simulink model "generate_joint_velocity_motion"  (R2019a)
settings: Solver=FixedStepDiscrete  StartTime=0.0  StopTime=inf  FixedStep=0.001  RelTol=1e-3  EnableMultiTasking=on
PreLoadFcn:
  | demos_common_configs();
undefined symbols (not defined in the file): DiscIntNeverNeededParam
libraries: franka_simulink_library_misc x5, franka_simulink_library x3
settings Model: SimulationMode=external  ExtModeTrigDuration=10000  Creator=vasi_ko  LastModifiedBy=kvasios
settings DataIOCC: LimitDataPoints=on  SaveFormat=Array  ReturnWorkspaceOutputs=off
settings OptimizationCC: DefaultParameterBehavior=Inlined  EnhancedBackFolding=on  PassReuseOutputArgsAs=Individual arguments  ZeroExternalMemoryAtStartup=off  ZeroInternalMemoryAtStartup=off  OptimizeBlockOrder=speed  DifferentSizesBufferReuse=on  OptimizationCustomize=off
settings DebuggingCC: SolverPrmCheckMsg=warning  ParameterTunabilityLossMsg=error  SFUnexpectedBacktrackingDiag=warning  SFNoUnconditionalDefaultTransitionDiag=warning  SFExecutionAtInitializationDiag=none  ArithmeticOperatorsInVariantConditions=warning
settings HardwareCC: ProdBitPerLong=64  ProdHWDeviceType=Intel->x86-64 (Linux 64)
settings ModelReferenceCC: PropagateSignalLabelsOutOfModel=off
settings SFSimCC: SimUseLocalCustomCode=off  MATLABDynamicMemAlloc=off
settings RTWCC: SystemTargetFile=franka_emika_panda.tlc  GenCodeOnly=on  TemplateMakefile=ert_default_tmf  RTWVerbose=off  RTWUseLocalCustomCode=off  Toolchain=Franka Simulink | gmake (64-bit linux)  BuildConfiguration=Faster Runs  IncludeHyperlinkInReport=on  TargetLang=C++
settings CodeAppCC: ForceParamTrailComments=on  IgnoreCustomStorageClasses=off  OperatorAnnotations=on  SimulinkDataObjDesc=on  SFDataObjDesc=on  InsertBlockDesc=on
settings STFCustomTargetCC: TargetLangStandard=C99 (ISO)  MultiwordLength=256  GenerateSampleERTMain=on  ModelReferenceCompliant=off  CombineOutputUpdateFcns=on  ERTCustomFileBanners=on  SupportNonInlinedSFcns=off  RemoveResetFunc=on  MATLABClassNameForMDSCustomization=Simulink.SoftwareTarget.ERTCustomization  CPPClassGenCompliant=on  GRTInterface=off  UseToolchainInfoCompliant=on  SystemTargetFile=franka_emika_panda.tlc
settings ERTTargetCC: TargetLangStandard=C99 (ISO)  GenerateSampleERTMain=on  ModelReferenceCompliant=off  ParMdlRefBuildCompliant=off  CompOptLevelCompliant=off  ConcurrentExecutionCompliant=off  SupportContinuousTime=on  ModelStepFunctionPrototypeControlCompliant=off  InlinedParameterPlacement=NonHierarchical  ERTCustomFileTemplate=franka_emika_panda_file_process.tlc
settings ConfigComp: CovMetricSettings=dw  CovSaveCumulativeToWorkspaceVar=on  CovSaveSingleToWorkspaceVar=on  CovExternalEMLEnable=off  CovSFcnEnable=off

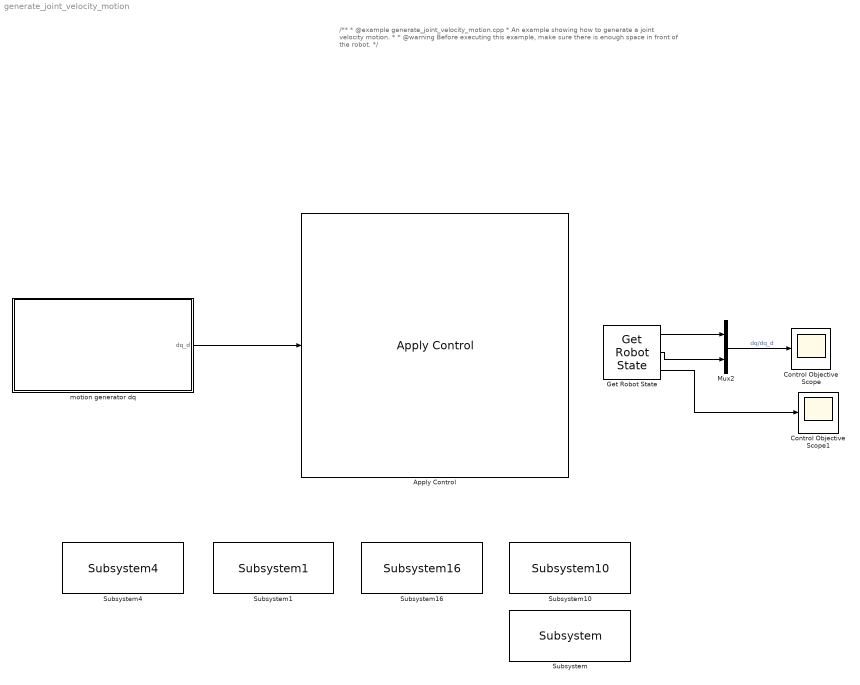
== system generate_joint_velocity_motion ==
  note: /**
      |  * @example generate_joint_velocity_motion.cpp
      |  * An example showing how to generate a joint velocity motion.
      |  *
      |  * @warning Before executing this example, make sure there is enough space in front of the robot.
      |  */
  Apply Control : franka_simulink_library/Apply Control  robot_ip=robot_ip  gripper_attached=off  control_mode=Joint Velocities - Internal Controller Mode  controller_choice=Joint Impedance Controller  elbow_control=on  collision_thresholds=collision_behavior  joint_impedance=joint_impedance  cartesian_impedance=cartesian_impedance  load_inertia=load_inertia  EE_T_K=EE_T_K  init_joint_configuration_req=on  init_joint_configuration=[0, -pi/4, 0, -3 * pi/4, 0, pi/2, pi/4]
      settings: SourceProductName=Franka Emika
  Control Objective Scope : Scope
  Control Objective Scope1 : Scope
  Get Robot State : franka_simulink_library/Get Robot State  robot_ip=robot_ip  signals_requested='dq dq_d control_command_success_rate'
      settings: SourceProductName=Franka Emika
  Mux2 : Mux  Inputs=2
  Subsystem : franka_simulink_library_misc/Subsystem  SystemSampleTime=-1  Latency=0  AutoFrameSizeCalculation=off
  Subsystem1 : franka_simulink_library_misc/Subsystem1  SystemSampleTime=-1  Latency=0  AutoFrameSizeCalculation=off
  Subsystem10 : franka_simulink_library_misc/Subsystem10  SystemSampleTime=-1  Latency=0  AutoFrameSizeCalculation=off
  Subsystem16 : franka_simulink_library_misc/Subsystem16  SystemSampleTime=-1  Latency=0  AutoFrameSizeCalculation=off
  Subsystem4 : franka_simulink_library_misc/Subsystem4  SystemSampleTime=-1  Latency=0  AutoFrameSizeCalculation=off
  motion generator dq : Subsystem
      mask Display:
      | pos = get_param(gcb, 'Position');
      | width = pos(3) - pos(1);
      | x = [0:width];
      | y = sin(x/180*pi);
      | % Parameters 'm' and 'b' must be defined in 'Parameters & Dialog' pane.
      | plot(x,y );
      | 
      | port_label('output',1,'dq_d');
  wires:
  Get Robot State/1 -> Mux2/1
  Get Robot State/2 -> Mux2/2
  Mux2/1 -> Control Objective Scope/1  "dq/dq_d"
  motion generator dq/1(dq_d) -> Apply Control/1
  Get Robot State/3 -> Control Objective Scope1/1

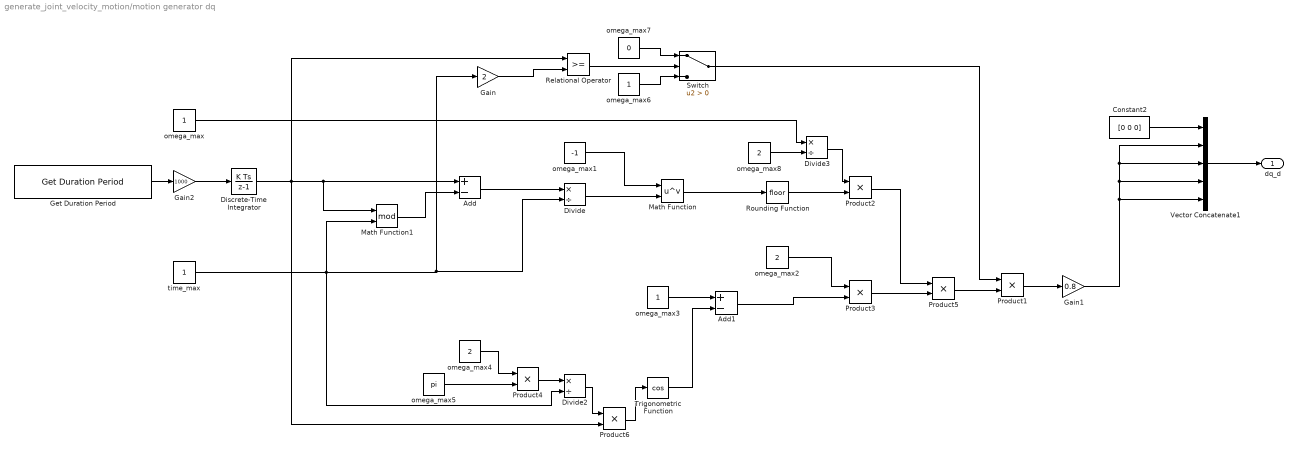
== system generate_joint_velocity_motion/motion generator dq ==
  Add : Sum  Inputs=+-
  Add1 : Sum  Inputs=+-
  Constant2 : Constant  Value=[0 0 0]  VectorParams1D=off
  Discrete-Time Integrator : DiscreteIntegrator  SampleTime=0.001  ICPrevOutput=DiscIntNeverNeededParam  ICPrevScaledInput=DiscIntNeverNeededParam
  Divide : Product  Inputs=*/
  Divide2 : Product  Inputs=*/
  Divide3 : Product  Inputs=*/
  Gain : Gain  Gain=2
  Gain1 : Gain  Gain=0.8
  Gain2 : Gain  Gain=1000
  Get Duration Period : franka_simulink_library/Get Duration Period  robot_ip=robot_ip
      settings: SourceProductName=Franka Emika
  Math Function : Math  Operator=pow  SaturateOnIntegerOverflow=on
  Math Function1 : Math  Operator=mod  SaturateOnIntegerOverflow=on
  Product{1..6} (6 alike) : Product
  Relational Operator : RelationalOperator  OutDataTypeStr=boolean  RndMeth=Nearest
  Rounding Function : Rounding
  Switch : Switch  Criteria=u2 > Threshold
  Trigonometric Function : Trigonometry  Operator=cos
  Vector Concatenate1 : Concatenate  NumInputs=5
  omega_max : Constant  VectorParams1D=off
  omega_max1 : Constant  Value=-1  VectorParams1D=off
  omega_max2 : Constant  Value=2  VectorParams1D=off
  omega_max3 : Constant  VectorParams1D=off
  omega_max4 : Constant  Value=2  VectorParams1D=off
  omega_max5 : Constant  Value=pi  VectorParams1D=off
  omega_max6 : Constant  VectorParams1D=off
  omega_max7 : Constant  Value=0  VectorParams1D=off
  omega_max8 : Constant  Value=2  VectorParams1D=off
  time_max : Constant  VectorParams1D=off
  dq_d : Outport  VectorParamsAs1DForOutWhenUnconnected=off
  wires:
  Product5/1 -> Product1/2
  Product3/1 -> Product5/2
  Product2/1 -> Product5/1
  Divide3/1 -> Product2/1
  omega_max8/1 -> Divide3/2
  Product6/1 -> Trigonometric Function/1
  Divide2/1 -> Product6/1
  Gain/1 -> Relational Operator/2
  omega_max7/1 -> Switch/1
  Switch/1 -> Product1/1
  omega_max6/1 -> Switch/3
  Relational Operator/1 -> Switch/2
  Constant2/1 -> Vector Concatenate1/1
  Gain2/1 -> Discrete-Time Integrator/1
  Vector Concatenate1/1 -> dq_d/1
  Discrete-Time Integrator/1 -> Add/1, Math Function1/1, Relational Operator/1, Product6/2
  time_max/1 -> Math Function1/2, Divide/2, Gain/1, Divide2/2
  Math Function1/1 -> Add/2
  Add/1 -> Divide/1
  Math Function/1 -> Rounding Function/1
  Divide/1 -> Math Function/2
  omega_max1/1 -> Math Function/1
  Rounding Function/1 -> Product2/2
  omega_max/1 -> Divide3/1
  omega_max2/1 -> Product3/1
  omega_max3/1 -> Add1/1
  omega_max4/1 -> Product4/1
  Add1/1 -> Product3/2
  Trigonometric Function/1 -> Add1/2
  Product4/1 -> Divide2/1
  omega_max5/1 -> Product4/2
  Product1/1 -> Gain1/1
  Gain1/1 -> Vector Concatenate1/5, Vector Concatenate1/4, Vector Concatenate1/3, Vector Concatenate1/2
  Get Duration Period/1 -> Gain2/1
